simulink model "SecRwRtStLgrstInwdOtwdTrgtPosSelc"  (R2018b)
settings: Solver=FixedStepDiscrete  StartTime=0.0  StopTime=10.0  FixedStep=0.01  RelTol=1e-3
undefined symbols (not defined in the file or in its folder): KeSMSw4SAcsMd24SecRwRtStLegrstOtwdInwdPos_Val, KeSMSw4SAcsMd24SecRwRtStLegrstOtwdInwdPosMax_Val, KeSMSw4SAcsMd24SecRwRtStLegrstOtwdInwdPosMin_Val, KeSMSw4SAcsMd26SecRwRtStLegrstOtwdInwdPos_Val, KeSMSw4SAcsMd26SecRwRtStLegrstOtwdInwdPosMax_Val, KeSMSw4SAcsMd26SecRwRtStLegrstOtwdInwdPosMin_Val, KeSMSw4SLegrstCloseMdSecRwRtStLgrstOtwdInwdPos_Val, KeSMSw4SLegrstCloseMdSecRwRtStLgrstOtwdInwdPosMax_Val, KeSMSw4SLegrstCloseMdSecRwRtStLgrstOtwdInwdPosMin_Val, KeSMSw4SLegrstOpenMdSecRwRtStLgrstOtwdInwdPos_Val, KeSMSw4SLegrstOpenMdSecRwRtStLgrstOtwdInwdPosMax_Val, KeSMSw4SLegrstOpenMdSecRwRtStLgrstOtwdInwdPosMin_Val, KeSMSw4sLyingMDSecRwRtStLgrstOtwdInwdPos_160_Val, KeSMSw4sLyingMDSecRwRtStLgrstOtwdInwdPos_165_Val, KeSMSw4sLyingMDSecRwRtStLgrstOtwdInwdPos_170_Val, KeSMSw4sLyingMDSecRwRtStLgrstOtwdInwdPos_175_Val, KeSMSw4sLyingMDSecRwRtStLgrstOtwdInwdPos_180_Val, KeSMSw4sLyingMDSecRwRtStLgrstOtwdInwdPos_Below160_Val, KeSMSw4sLyingMDSecRwRtStLgrstOtwdInwdPos_Over180_Val, KeSMSw4sLyingMDSecRwRtStLgrstOtwdInwdPosMax_160_Val, KeSMSw4sLyingMDSecRwRtStLgrstOtwdInwdPosMax_165_Val, KeSMSw4sLyingMDSecRwRtStLgrstOtwdInwdPosMax_170_Val, KeSMSw4sLyingMDSecRwRtStLgrstOtwdInwdPosMax_175_Val, KeSMSw4sLyingMDSecRwRtStLgrstOtwdInwdPosMax_180_Val, KeSMSw4sLyingMDSecRwRtStLgrstOtwdInwdPosMax_Below160_Val, KeSMSw4sLyingMDSecRwRtStLgrstOtwdInwdPosMax_Over180_Val, KeSMSw4sLyingMDSecRwRtStLgrstOtwdInwdPosMin_160_Val, KeSMSw4sLyingMDSecRwRtStLgrstOtwdInwdPosMin_165_Val, KeSMSw4sLyingMDSecRwRtStLgrstOtwdInwdPosMin_170_Val, KeSMSw4sLyingMDSecRwRtStLgrstOtwdInwdPosMin_175_Val, KeSMSw4sLyingMDSecRwRtStLgrstOtwdInwdPosMin_180_Val, KeSMSw4sLyingMDSecRwRtStLgrstOtwdInwdPosMin_Below160_Val, KeSMSw4sLyingMDSecRwRtStLgrstOtwdInwdPosMin_Over180_Val, KeSMSw4sRecoveryMDSecRwRtStLgrstOtwdInwdPos_160_Val, KeSMSw4sRecoveryMDSecRwRtStLgrstOtwdInwdPos_165_Val, KeSMSw4sRecoveryMDSecRwRtStLgrstOtwdInwdPos_170_Val, KeSMSw4sRecoveryMDSecRwRtStLgrstOtwdInwdPos_175_Val, KeSMSw4sRecoveryMDSecRwRtStLgrstOtwdInwdPos_180_Val, KeSMSw4sRecoveryMDSecRwRtStLgrstOtwdInwdPos_Below160_Val, KeSMSw4sRecoveryMDSecRwRtStLgrstOtwdInwdPos_Over180_Val, KeSMSw4sRecoveryMDSecRwRtStLgrstOtwdInwdPosMax_160_Val, KeSMSw4sRecoveryMDSecRwRtStLgrstOtwdInwdPosMax_165_Val, KeSMSw4sRecoveryMDSecRwRtStLgrstOtwdInwdPosMax_170_Val, KeSMSw4sRecoveryMDSecRwRtStLgrstOtwdInwdPosMax_175_Val, KeSMSw4sRecoveryMDSecRwRtStLgrstOtwdInwdPosMax_180_Val, KeSMSw4sRecoveryMDSecRwRtStLgrstOtwdInwdPosMax_Below160_Val, KeSMSw4sRecoveryMDSecRwRtStLgrstOtwdInwdPosMax_Over180_Val, KeSMSw4sRecoveryMDSecRwRtStLgrstOtwdInwdPosMin_160_Val, KeSMSw4sRecoveryMDSecRwRtStLgrstOtwdInwdPosMin_165_Val, KeSMSw4sRecoveryMDSecRwRtStLgrstOtwdInwdPosMin_170_Val, KeSMSw4sRecoveryMDSecRwRtStLgrstOtwdInwdPosMin_175_Val, KeSMSw4sRecoveryMDSecRwRtStLgrstOtwdInwdPosMin_180_Val, KeSMSw4sRecoveryMDSecRwRtStLgrstOtwdInwdPosMin_Below160_Val, KeSMSw4sRecoveryMDSecRwRtStLgrstOtwdInwdPosMin_Over180_Val, KeSMSw4sVIPMDSecRwRtStLgrstOtwdInwdPos_160_Val, KeSMSw4sVIPMDSecRwRtStLgrstOtwdInwdPos_165_Val, KeSMSw4sVIPMDSecRwRtStLgrstOtwdInwdPos_170_Val, KeSMSw4sVIPMDSecRwRtStLgrstOtwdInwdPos_175_Val, KeSMSw4sVIPMDSecRwRtStLgrstOtwdInwdPos_180_Val, KeSMSw4sVIPMDSecRwRtStLgrstOtwdInwdPos_Below160_Val ... (+40)
libraries: TrgtPosSelcLib x10
(part 1 of 2)
settings Model: Creator=sn2xws  LastModifiedBy=sn2xws
settings Model: ModifiedHistory=|
  | 2023.8.1 V2.0.0 CR401790 增加模式21-26
  | 2024.5.6 V3.0.0 557 67座增加腿托延伸
  | 2024.7.9 V3.0.1557模式流程V1.9
settings DataIOCC: SaveFormat=StructureWithTime
settings OptimizationCC: DefaultParameterBehavior=Inlined  EnhancedBackFolding=on  PassReuseOutputArgsAs=Individual arguments  ZeroExternalMemoryAtStartup=off  ZeroInternalMemoryAtStartup=off  OptimizeBlockOrder=speed  DifferentSizesBufferReuse=on  OptimizationCustomize=off
settings DebuggingCC: ParameterTunabilityLossMsg=error
settings ModelReferenceCC: ModelReferenceNumInstancesAllowed=Single
settings SFSimCC: MATLABDynamicMemAlloc=off
settings RTWCC: SystemTargetFile=autosar.tlc  GenCodeOnly=on  TemplateMakefile=ert_default_tmf  Description=AUTOSAR  GenerateReport=on  IncludeHyperlinkInReport=on  LaunchReport=on  GenerateTraceInfo=on  GenerateTraceReport=on  GenerateTraceReportSl=on  GenerateTraceReportSf=on  GenerateTraceReportEml=on
settings CodeAppCC: ForceParamTrailComments=on  IgnoreCustomStorageClasses=off  OperatorAnnotations=on  SimulinkDataObjDesc=on  SFDataObjDesc=on  InsertBlockDesc=on
settings STFCustomTargetCC: TargetLangStandard=C99 (ISO)  MultiwordLength=256  ParMdlRefBuildCompliant=on  CompOptLevelCompliant=on  IncludeMdlTerminateFcn=off  CombineOutputUpdateFcns=on  SuppressErrorStatus=on  ERTCustomFileBanners=on  SupportNonFinite=off  SupportComplex=off  SupportContinuousTime=off  SupportNonInlinedSFcns=off  RemoveResetFunc=on  MATLABClassNameForMDSCustomization=Simulink.SoftwareTarget.ERTCustomization  AutosarCompliant=on  UseToolchainInfoCompliant=on  LookupTableObjectStructAxisOrder=2,1,3,4,...  LUTObjectStructOrderEvenSpacing=Size,Table,Breakpoints  SystemTargetFile=autosar.tlc
settings ERTTargetCC: TargetLangStandard=C99 (ISO)  ConcurrentExecutionCompliant=off  IncludeMdlTerminateFcn=off  SuppressErrorStatus=on  SupportNonFinite=off  SupportComplex=off  ModelStepFunctionPrototypeControlCompliant=off  CPPClassGenCompliant=off  AutosarCompliant=on  LookupTableObjectStructAxisOrder=2,1,3,4,...  LUTObjectStructOrderEvenSpacing=Size,Table,Breakpoints  InlinedParameterPlacement=NonHierarchical  ERTCustomFileTemplate=example_file_process.tlc  ERTFilePackagingFormat=Compact

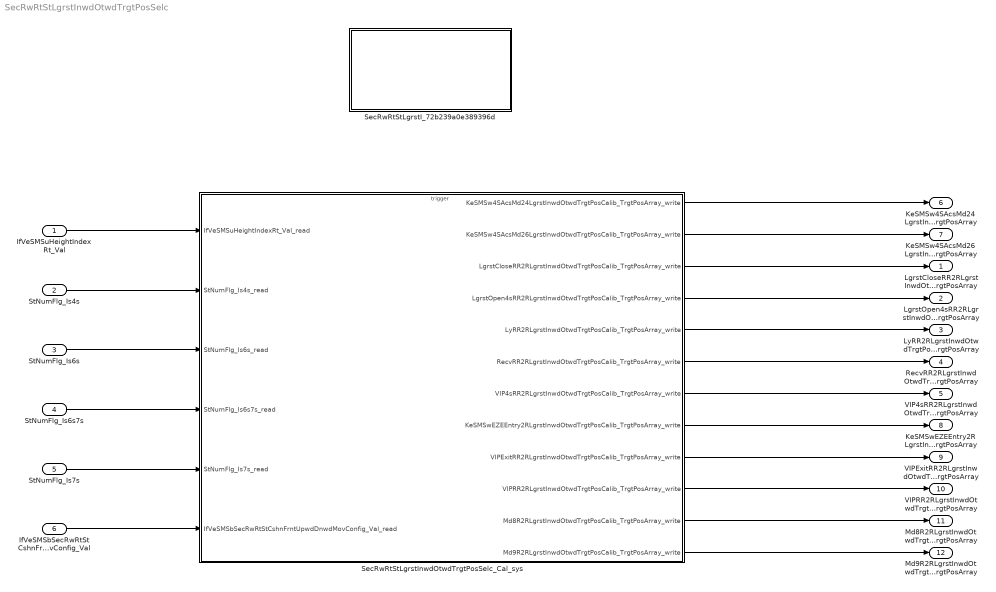
== system SecRwRtStLgrstInwdOtwdTrgtPosSelc ==
  IfVeSMSuHeightIndexRt_Val : Inport  Description=|  OutDataTypeStr=uint8  PortDimensions=1
      | 0：under 160
      | 1：160
      | 2：165
      | 3：170
      | 4：175
      | 5：180
      | 6：over 180
  StNumFlg_Is4s : Inport  Port=2  OutDataTypeStr=boolean  PortDimensions=1
  StNumFlg_Is6s : Inport  Port=3  OutDataTypeStr=boolean  PortDimensions=1
  StNumFlg_Is6s7s : Inport  Port=4  OutDataTypeStr=boolean  PortDimensions=1
  StNumFlg_Is7s : Inport  Port=5  OutDataTypeStr=boolean  PortDimensions=1
  IfVeSMSbSecRwRtStCshnFrntUpwdDnwdMovConfig_Val : Inport  Port=6  OutDataTypeStr=boolean  PortDimensions=1
  SecRwRtStLgrstI_72b239a0e389396d : Subsystem
  SecRwRtStLgrstInwdOtwdTrgtPosSelc_Cal_sys : Subsystem
  LgrstCloseRR2RLgrstInwdOtwdTrgtPosCalib_TrgtPosArray : Outport  Description=|  OutDataTypeStr=uint16  PortDimensions=3
      | 0:Pos
      | 1:Max
      | 2:Min
  LgrstOpen4sRR2RLgrstInwdOtwdTrgtPosCalib_TrgtPosArray : Outport  Description=|  Port=2  OutDataTypeStr=uint16  PortDimensions=3
      | 0:Pos
      | 1:Max
      | 2:Min
  LyRR2RLgrstInwdOtwdTrgtPosCalib_TrgtPosArray : Outport  Description=|  Port=3  OutDataTypeStr=uint16  PortDimensions=3
      | 0:Pos
      | 1:Max
      | 2:Min
  RecvRR2RLgrstInwdOtwdTrgtPosCalib_TrgtPosArray : Outport  Description=|  Port=4  OutDataTypeStr=uint16  PortDimensions=3
      | 0:Pos
      | 1:Max
      | 2:Min
  VIP4sRR2RLgrstInwdOtwdTrgtPosCalib_TrgtPosArray : Outport  Description=|  Port=5  OutDataTypeStr=uint16  PortDimensions=3
      | 0:Pos
      | 1:Max
      | 2:Min
  KeSMSw4SAcsMd24LgrstInwdOtwdTrgtPosCalib_TrgtPosArray : Outport  Description=|  Port=6  OutDataTypeStr=uint16  PortDimensions=3
      | 0:Pos
      | 1:Max
      | 2:Min
  KeSMSw4SAcsMd26LgrstInwdOtwdTrgtPosCalib_TrgtPosArray : Outport  Description=|  Port=7  OutDataTypeStr=uint16  PortDimensions=3
      | 0:Pos
      | 1:Max
      | 2:Min
  KeSMSwEZEEntry2RLgrstInwdOtwdTrgtPosCalib_TrgtPosArray : Outport  Description=|  Port=8  OutDataTypeStr=uint16  PortDimensions=3
      | 0:Pos
      | 1:Max
      | 2:Min
  VIPExitRR2RLgrstInwdOtwdTrgtPosCalib_TrgtPosArray : Outport  Description=|  Port=9  OutDataTypeStr=uint16  PortDimensions=3
      | 0:Pos
      | 1:Max
      | 2:Min
  VIPRR2RLgrstInwdOtwdTrgtPosCalib_TrgtPosArray : Outport  Description=|  Port=10  OutDataTypeStr=uint16  PortDimensions=3
      | 0:Pos
      | 1:Max
      | 2:Min
  Md8R2RLgrstInwdOtwdTrgtPosCalib_TrgtPosArray : Outport  Description=|  Port=11  OutDataTypeStr=uint16  PortDimensions=3
      | 0:Pos
      | 1:Max
      | 2:Min
  Md9R2RLgrstInwdOtwdTrgtPosCalib_TrgtPosArray : Outport  Description=|  Port=12  OutDataTypeStr=uint16  PortDimensions=3
      | 0:Pos
      | 1:Max
      | 2:Min
  wires:
  IfVeSMSuHeightIndexRt_Val/1 -> SecRwRtStLgrstInwdOtwdTrgtPosSelc_Cal_sys/1(IfVeSMSuHeightIndexRt_Val_read)
  StNumFlg_Is4s/1 -> SecRwRtStLgrstInwdOtwdTrgtPosSelc_Cal_sys/2(StNumFlg_Is4s_read)
  StNumFlg_Is6s/1 -> SecRwRtStLgrstInwdOtwdTrgtPosSelc_Cal_sys/3(StNumFlg_Is6s_read)
  StNumFlg_Is6s7s/1 -> SecRwRtStLgrstInwdOtwdTrgtPosSelc_Cal_sys/4(StNumFlg_Is6s7s_read)
  StNumFlg_Is7s/1 -> SecRwRtStLgrstInwdOtwdTrgtPosSelc_Cal_sys/5(StNumFlg_Is7s_read)
  SecRwRtStLgrstInwdOtwdTrgtPosSelc_Cal_sys/3(LgrstCloseRR2RLgrstInwdOtwdTrgtPosCalib_TrgtPosArray_write) -> LgrstCloseRR2RLgrstInwdOtwdTrgtPosCalib_TrgtPosArray/1
  SecRwRtStLgrstInwdOtwdTrgtPosSelc_Cal_sys/4(LgrstOpen4sRR2RLgrstInwdOtwdTrgtPosCalib_TrgtPosArray_write) -> LgrstOpen4sRR2RLgrstInwdOtwdTrgtPosCalib_TrgtPosArray/1
  SecRwRtStLgrstInwdOtwdTrgtPosSelc_Cal_sys/5(LyRR2RLgrstInwdOtwdTrgtPosCalib_TrgtPosArray_write) -> LyRR2RLgrstInwdOtwdTrgtPosCalib_TrgtPosArray/1
  SecRwRtStLgrstInwdOtwdTrgtPosSelc_Cal_sys/6(RecvRR2RLgrstInwdOtwdTrgtPosCalib_TrgtPosArray_write) -> RecvRR2RLgrstInwdOtwdTrgtPosCalib_TrgtPosArray/1
  SecRwRtStLgrstInwdOtwdTrgtPosSelc_Cal_sys/7(VIP4sRR2RLgrstInwdOtwdTrgtPosCalib_TrgtPosArray_write) -> VIP4sRR2RLgrstInwdOtwdTrgtPosCalib_TrgtPosArray/1
  SecRwRtStLgrstInwdOtwdTrgtPosSelc_Cal_sys/1(KeSMSw4SAcsMd24LgrstInwdOtwdTrgtPosCalib_TrgtPosArray_write) -> KeSMSw4SAcsMd24LgrstInwdOtwdTrgtPosCalib_TrgtPosArray/1
  SecRwRtStLgrstInwdOtwdTrgtPosSelc_Cal_sys/2(KeSMSw4SAcsMd26LgrstInwdOtwdTrgtPosCalib_TrgtPosArray_write) -> KeSMSw4SAcsMd26LgrstInwdOtwdTrgtPosCalib_TrgtPosArray/1
  SecRwRtStLgrstInwdOtwdTrgtPosSelc_Cal_sys/8(KeSMSwEZEEntry2RLgrstInwdOtwdTrgtPosCalib_TrgtPosArray_write) -> KeSMSwEZEEntry2RLgrstInwdOtwdTrgtPosCalib_TrgtPosArray/1
  IfVeSMSbSecRwRtStCshnFrntUpwdDnwdMovConfig_Val/1 -> SecRwRtStLgrstInwdOtwdTrgtPosSelc_Cal_sys/6(IfVeSMSbSecRwRtStCshnFrntUpwdDnwdMovConfig_Val_read)
  SecRwRtStLgrstInwdOtwdTrgtPosSelc_Cal_sys/9(VIPExitRR2RLgrstInwdOtwdTrgtPosCalib_TrgtPosArray_write) -> VIPExitRR2RLgrstInwdOtwdTrgtPosCalib_TrgtPosArray/1
  SecRwRtStLgrstInwdOtwdTrgtPosSelc_Cal_sys/10(VIPRR2RLgrstInwdOtwdTrgtPosCalib_TrgtPosArray_write) -> VIPRR2RLgrstInwdOtwdTrgtPosCalib_TrgtPosArray/1
  SecRwRtStLgrstInwdOtwdTrgtPosSelc_Cal_sys/11(Md8R2RLgrstInwdOtwdTrgtPosCalib_TrgtPosArray_write) -> Md8R2RLgrstInwdOtwdTrgtPosCalib_TrgtPosArray/1
  SecRwRtStLgrstInwdOtwdTrgtPosSelc_Cal_sys/12(Md9R2RLgrstInwdOtwdTrgtPosCalib_TrgtPosArray_write) -> Md9R2RLgrstInwdOtwdTrgtPosCalib_TrgtPosArray/1

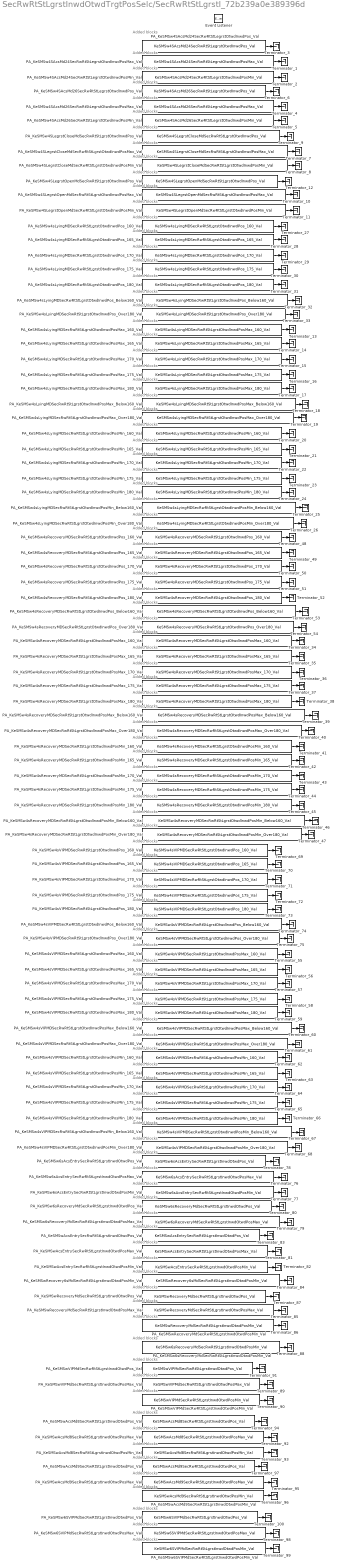
== system SecRwRtStLgrstInwdOtwdTrgtPosSelc/SecRwRtStLgrstI_72b239a0e389396d ==
  note: Added blocks
  note: Added blocks
  note: Added blocks
  note: Added blocks
  note: Added blocks
  note: Added blocks
  note: Added blocks
  note: Added blocks
  note: Added blocks
  note: Added blocks
  note: Added blocks
  note: Added blocks
  note: Added blocks
  note: Added blocks
  note: Added blocks
  note: Added blocks
  note: Added blocks
  note: Added blocks
  note: Added blocks
  note: Added blocks
  note: Added blocks
  note: Added blocks
  note: Added blocks
  note: Added blocks
  note: Added blocks
  note: Added blocks
  note: Added blocks
  note: Added blocks
  note: Added blocks
  note: Added blocks
  note: Added blocks
  note: Added blocks
  note: Added blocks
  note: Added blocks
  note: Added blocks
  note: Added blocks
  note: Added blocks
  note: Added blocks
  note: Added blocks
  note: Added blocks
  note: Added blocks
  note: Added blocks
  note: Added blocks
  note: Added blocks
  note: Added blocks
  note: Added blocks
  note: Added blocks
  note: Added blocks
  note: Added blocks
  note: Added blocks
  note: Added blocks
  note: Added blocks
  note: Added blocks
  note: Added blocks
  note: Added blocks
  note: Added blocks
  note: Added blocks
  note: Added blocks
  note: Added blocks
  note: Added blocks
  note: Added blocks
  note: Added blocks
  note: Added blocks
  note: Added blocks
  note: Added blocks
  note: Added blocks
  note: Added blocks
  note: Added blocks
  note: Added blocks
  note: Added blocks
  note: Added blocks
  note: Added blocks
  note: Added blocks
  note: Added blocks
  note: Added blocks
  note: Added blocks
  note: Added blocks
  note: Added blocks
  note: Added blocks
  note: Added blocks
  note: Added blocks
  note: Added blocks
  note: Added blocks
  note: Added blocks
  note: Added blocks
  note: Added blocks
  note: Added blocks
  note: Added blocks
  note: Added blocks
  note: Added blocks
  note: Added blocks
  note: Added blocks
  note: Added blocks
  note: Added blocks
  note: Added blocks
  note: Added blocks
  note: Added blocks
  note: Added blocks
  note: Added blocks
  note: Added blocks
  Event Listener : EventListener  EventName=reset
  PA_KeSMSw4SAcsMd24SecRwRtStLegrstOtwdInwdPosMax_Val : Constant  Value=KeSMSw4SAcsMd24SecRwRtStLegrstOtwdInwdPosMax_Val
  PA_KeSMSw4SAcsMd24SecRwRtStLegrstOtwdInwdPosMin_Val : Constant  Value=KeSMSw4SAcsMd24SecRwRtStLegrstOtwdInwdPosMin_Val
  PA_KeSMSw4SAcsMd24SecRwRtStLegrstOtwdInwdPos_Val : Constant  Value=KeSMSw4SAcsMd24SecRwRtStLegrstOtwdInwdPos_Val
  PA_KeSMSw4SAcsMd26SecRwRtStLegrstOtwdInwdPosMax_Val : Constant  Value=KeSMSw4SAcsMd26SecRwRtStLegrstOtwdInwdPosMax_Val
  PA_KeSMSw4SAcsMd26SecRwRtStLegrstOtwdInwdPosMin_Val : Constant  Value=KeSMSw4SAcsMd26SecRwRtStLegrstOtwdInwdPosMin_Val
  PA_KeSMSw4SAcsMd26SecRwRtStLegrstOtwdInwdPos_Val : Constant  Value=KeSMSw4SAcsMd26SecRwRtStLegrstOtwdInwdPos_Val
  PA_KeSMSw4SLegrstCloseMdSecRwRtStLgrstOtwdInwdPosMax_Val : Constant  Value=KeSMSw4SLegrstCloseMdSecRwRtStLgrstOtwdInwdPosMax_Val
  PA_KeSMSw4SLegrstCloseMdSecRwRtStLgrstOtwdInwdPosMin_Val : Constant  Value=KeSMSw4SLegrstCloseMdSecRwRtStLgrstOtwdInwdPosMin_Val
  PA_KeSMSw4SLegrstCloseMdSecRwRtStLgrstOtwdInwdPos_Val : Constant  Value=KeSMSw4SLegrstCloseMdSecRwRtStLgrstOtwdInwdPos_Val
  PA_KeSMSw4SLegrstOpenMdSecRwRtStLgrstOtwdInwdPosMax_Val : Constant  Value=KeSMSw4SLegrstOpenMdSecRwRtStLgrstOtwdInwdPosMax_Val
  PA_KeSMSw4SLegrstOpenMdSecRwRtStLgrstOtwdInwdPosMin_Val : Constant  Value=KeSMSw4SLegrstOpenMdSecRwRtStLgrstOtwdInwdPosMin_Val
  PA_KeSMSw4SLegrstOpenMdSecRwRtStLgrstOtwdInwdPos_Val : Constant  Value=KeSMSw4SLegrstOpenMdSecRwRtStLgrstOtwdInwdPos_Val
  PA_KeSMSw4sLyingMDSecRwRtStLgrstOtwdInwdPosMax_160_Val : Constant  Value=KeSMSw4sLyingMDSecRwRtStLgrstOtwdInwdPosMax_160_Val
  PA_KeSMSw4sLyingMDSecRwRtStLgrstOtwdInwdPosMax_165_Val : Constant  Value=KeSMSw4sLyingMDSecRwRtStLgrstOtwdInwdPosMax_165_Val
  PA_KeSMSw4sLyingMDSecRwRtStLgrstOtwdInwdPosMax_170_Val : Constant  Value=KeSMSw4sLyingMDSecRwRtStLgrstOtwdInwdPosMax_170_Val
  PA_KeSMSw4sLyingMDSecRwRtStLgrstOtwdInwdPosMax_175_Val : Constant  Value=KeSMSw4sLyingMDSecRwRtStLgrstOtwdInwdPosMax_175_Val
  PA_KeSMSw4sLyingMDSecRwRtStLgrstOtwdInwdPosMax_180_Val : Constant  Value=KeSMSw4sLyingMDSecRwRtStLgrstOtwdInwdPosMax_180_Val
  PA_KeSMSw4sLyingMDSecRwRtStLgrstOtwdInwdPosMax_Below160_Val : Constant  Value=KeSMSw4sLyingMDSecRwRtStLgrstOtwdInwdPosMax_Below160_Val
  PA_KeSMSw4sLyingMDSecRwRtStLgrstOtwdInwdPosMax_Over180_Val : Constant  Value=KeSMSw4sLyingMDSecRwRtStLgrstOtwdInwdPosMax_Over180_Val
  PA_KeSMSw4sLyingMDSecRwRtStLgrstOtwdInwdPosMin_160_Val : Constant  Value=KeSMSw4sLyingMDSecRwRtStLgrstOtwdInwdPosMin_160_Val
  PA_KeSMSw4sLyingMDSecRwRtStLgrstOtwdInwdPosMin_165_Val : Constant  Value=KeSMSw4sLyingMDSecRwRtStLgrstOtwdInwdPosMin_165_Val
  PA_KeSMSw4sLyingMDSecRwRtStLgrstOtwdInwdPosMin_170_Val : Constant  Value=KeSMSw4sLyingMDSecRwRtStLgrstOtwdInwdPosMin_170_Val
  PA_KeSMSw4sLyingMDSecRwRtStLgrstOtwdInwdPosMin_175_Val : Constant  Value=KeSMSw4sLyingMDSecRwRtStLgrstOtwdInwdPosMin_175_Val
  PA_KeSMSw4sLyingMDSecRwRtStLgrstOtwdInwdPosMin_180_Val : Constant  Value=KeSMSw4sLyingMDSecRwRtStLgrstOtwdInwdPosMin_180_Val
  PA_KeSMSw4sLyingMDSecRwRtStLgrstOtwdInwdPosMin_Below160_Val : Constant  Value=KeSMSw4sLyingMDSecRwRtStLgrstOtwdInwdPosMin_Below160_Val
  PA_KeSMSw4sLyingMDSecRwRtStLgrstOtwdInwdPosMin_Over180_Val : Constant  Value=KeSMSw4sLyingMDSecRwRtStLgrstOtwdInwdPosMin_Over180_Val
  PA_KeSMSw4sLyingMDSecRwRtStLgrstOtwdInwdPos_160_Val : Constant  Value=KeSMSw4sLyingMDSecRwRtStLgrstOtwdInwdPos_160_Val
  PA_KeSMSw4sLyingMDSecRwRtStLgrstOtwdInwdPos_165_Val : Constant  Value=KeSMSw4sLyingMDSecRwRtStLgrstOtwdInwdPos_165_Val
  PA_KeSMSw4sLyingMDSecRwRtStLgrstOtwdInwdPos_170_Val : Constant  Value=KeSMSw4sLyingMDSecRwRtStLgrstOtwdInwdPos_170_Val
  PA_KeSMSw4sLyingMDSecRwRtStLgrstOtwdInwdPos_175_Val : Constant  Value=KeSMSw4sLyingMDSecRwRtStLgrstOtwdInwdPos_175_Val
  PA_KeSMSw4sLyingMDSecRwRtStLgrstOtwdInwdPos_180_Val : Constant  Value=KeSMSw4sLyingMDSecRwRtStLgrstOtwdInwdPos_180_Val
  PA_KeSMSw4sLyingMDSecRwRtStLgrstOtwdInwdPos_Below160_Val : Constant  Value=KeSMSw4sLyingMDSecRwRtStLgrstOtwdInwdPos_Below160_Val
  PA_KeSMSw4sLyingMDSecRwRtStLgrstOtwdInwdPos_Over180_Val : Constant  Value=KeSMSw4sLyingMDSecRwRtStLgrstOtwdInwdPos_Over180_Val
  PA_KeSMSw4sRecoveryMDSecRwRtStLgrstOtwdInwdPosMax_160_Val : Constant  Value=KeSMSw4sRecoveryMDSecRwRtStLgrstOtwdInwdPosMax_160_Val
  PA_KeSMSw4sRecoveryMDSecRwRtStLgrstOtwdInwdPosMax_165_Val : Constant  Value=KeSMSw4sRecoveryMDSecRwRtStLgrstOtwdInwdPosMax_165_Val
  PA_KeSMSw4sRecoveryMDSecRwRtStLgrstOtwdInwdPosMax_170_Val : Constant  Value=KeSMSw4sRecoveryMDSecRwRtStLgrstOtwdInwdPosMax_170_Val
  PA_KeSMSw4sRecoveryMDSecRwRtStLgrstOtwdInwdPosMax_175_Val : Constant  Value=KeSMSw4sRecoveryMDSecRwRtStLgrstOtwdInwdPosMax_175_Val
  PA_KeSMSw4sRecoveryMDSecRwRtStLgrstOtwdInwdPosMax_180_Val : Constant  Value=KeSMSw4sRecoveryMDSecRwRtStLgrstOtwdInwdPosMax_180_Val
  PA_KeSMSw4sRecoveryMDSecRwRtStLgrstOtwdInwdPosMax_Below160_Val : Constant  Value=KeSMSw4sRecoveryMDSecRwRtStLgrstOtwdInwdPosMax_Below160_Val
  PA_KeSMSw4sRecoveryMDSecRwRtStLgrstOtwdInwdPosMax_Over180_Val : Constant  Value=KeSMSw4sRecoveryMDSecRwRtStLgrstOtwdInwdPosMax_Over180_Val
  PA_KeSMSw4sRecoveryMDSecRwRtStLgrstOtwdInwdPosMin_160_Val : Constant  Value=KeSMSw4sRecoveryMDSecRwRtStLgrstOtwdInwdPosMin_160_Val
  PA_KeSMSw4sRecoveryMDSecRwRtStLgrstOtwdInwdPosMin_165_Val : Constant  Value=KeSMSw4sRecoveryMDSecRwRtStLgrstOtwdInwdPosMin_165_Val
  PA_KeSMSw4sRecoveryMDSecRwRtStLgrstOtwdInwdPosMin_170_Val : Constant  Value=KeSMSw4sRecoveryMDSecRwRtStLgrstOtwdInwdPosMin_170_Val
  PA_KeSMSw4sRecoveryMDSecRwRtStLgrstOtwdInwdPosMin_175_Val : Constant  Value=KeSMSw4sRecoveryMDSecRwRtStLgrstOtwdInwdPosMin_175_Val
  PA_KeSMSw4sRecoveryMDSecRwRtStLgrstOtwdInwdPosMin_180_Val : Constant  Value=KeSMSw4sRecoveryMDSecRwRtStLgrstOtwdInwdPosMin_180_Val
  PA_KeSMSw4sRecoveryMDSecRwRtStLgrstOtwdInwdPosMin_Below160_Val : Constant  Value=KeSMSw4sRecoveryMDSecRwRtStLgrstOtwdInwdPosMin_Below160_Val
  PA_KeSMSw4sRecoveryMDSecRwRtStLgrstOtwdInwdPosMin_Over180_Val : Constant  Value=KeSMSw4sRecoveryMDSecRwRtStLgrstOtwdInwdPosMin_Over180_Val
  PA_KeSMSw4sRecoveryMDSecRwRtStLgrstOtwdInwdPos_160_Val : Constant  Value=KeSMSw4sRecoveryMDSecRwRtStLgrstOtwdInwdPos_160_Val
  PA_KeSMSw4sRecoveryMDSecRwRtStLgrstOtwdInwdPos_165_Val : Constant  Value=KeSMSw4sRecoveryMDSecRwRtStLgrstOtwdInwdPos_165_Val
  PA_KeSMSw4sRecoveryMDSecRwRtStLgrstOtwdInwdPos_170_Val : Constant  Value=KeSMSw4sRecoveryMDSecRwRtStLgrstOtwdInwdPos_170_Val
  PA_KeSMSw4sRecoveryMDSecRwRtStLgrstOtwdInwdPos_175_Val : Constant  Value=KeSMSw4sRecoveryMDSecRwRtStLgrstOtwdInwdPos_175_Val
  PA_KeSMSw4sRecoveryMDSecRwRtStLgrstOtwdInwdPos_180_Val : Constant  Value=KeSMSw4sRecoveryMDSecRwRtStLgrstOtwdInwdPos_180_Val
  PA_KeSMSw4sRecoveryMDSecRwRtStLgrstOtwdInwdPos_Below160_Val : Constant  Value=KeSMSw4sRecoveryMDSecRwRtStLgrstOtwdInwdPos_Below160_Val
  PA_KeSMSw4sRecoveryMDSecRwRtStLgrstOtwdInwdPos_Over180_Val : Constant  Value=KeSMSw4sRecoveryMDSecRwRtStLgrstOtwdInwdPos_Over180_Val
  PA_KeSMSw4sVIPMDSecRwRtStLgrstOtwdInwdPosMax_160_Val : Constant  Value=KeSMSw4sVIPMDSecRwRtStLgrstOtwdInwdPosMax_160_Val
  PA_KeSMSw4sVIPMDSecRwRtStLgrstOtwdInwdPosMax_165_Val : Constant  Value=KeSMSw4sVIPMDSecRwRtStLgrstOtwdInwdPosMax_165_Val
  PA_KeSMSw4sVIPMDSecRwRtStLgrstOtwdInwdPosMax_170_Val : Constant  Value=KeSMSw4sVIPMDSecRwRtStLgrstOtwdInwdPosMax_170_Val
  PA_KeSMSw4sVIPMDSecRwRtStLgrstOtwdInwdPosMax_175_Val : Constant  Value=KeSMSw4sVIPMDSecRwRtStLgrstOtwdInwdPosMax_175_Val
  PA_KeSMSw4sVIPMDSecRwRtStLgrstOtwdInwdPosMax_180_Val : Constant  Value=KeSMSw4sVIPMDSecRwRtStLgrstOtwdInwdPosMax_180_Val
  PA_KeSMSw4sVIPMDSecRwRtStLgrstOtwdInwdPosMax_Below160_Val : Constant  Value=KeSMSw4sVIPMDSecRwRtStLgrstOtwdInwdPosMax_Below160_Val
  PA_KeSMSw4sVIPMDSecRwRtStLgrstOtwdInwdPosMax_Over180_Val : Constant  Value=KeSMSw4sVIPMDSecRwRtStLgrstOtwdInwdPosMax_Over180_Val
  PA_KeSMSw4sVIPMDSecRwRtStLgrstOtwdInwdPosMin_160_Val : Constant  Value=KeSMSw4sVIPMDSecRwRtStLgrstOtwdInwdPosMin_160_Val
  PA_KeSMSw4sVIPMDSecRwRtStLgrstOtwdInwdPosMin_165_Val : Constant  Value=KeSMSw4sVIPMDSecRwRtStLgrstOtwdInwdPosMin_165_Val
  PA_KeSMSw4sVIPMDSecRwRtStLgrstOtwdInwdPosMin_170_Val : Constant  Value=KeSMSw4sVIPMDSecRwRtStLgrstOtwdInwdPosMin_170_Val
  PA_KeSMSw4sVIPMDSecRwRtStLgrstOtwdInwdPosMin_175_Val : Constant  Value=KeSMSw4sVIPMDSecRwRtStLgrstOtwdInwdPosMin_175_Val
  PA_KeSMSw4sVIPMDSecRwRtStLgrstOtwdInwdPosMin_180_Val : Constant  Value=KeSMSw4sVIPMDSecRwRtStLgrstOtwdInwdPosMin_180_Val
  PA_KeSMSw4sVIPMDSecRwRtStLgrstOtwdInwdPosMin_Below160_Val : Constant  Value=KeSMSw4sVIPMDSecRwRtStLgrstOtwdInwdPosMin_Below160_Val
  PA_KeSMSw4sVIPMDSecRwRtStLgrstOtwdInwdPosMin_Over180_Val : Constant  Value=KeSMSw4sVIPMDSecRwRtStLgrstOtwdInwdPosMin_Over180_Val
  PA_KeSMSw4sVIPMDSecRwRtStLgrstOtwdInwdPos_160_Val : Constant  Value=KeSMSw4sVIPMDSecRwRtStLgrstOtwdInwdPos_160_Val
  PA_KeSMSw4sVIPMDSecRwRtStLgrstOtwdInwdPos_165_Val : Constant  Value=KeSMSw4sVIPMDSecRwRtStLgrstOtwdInwdPos_165_Val
  PA_KeSMSw4sVIPMDSecRwRtStLgrstOtwdInwdPos_170_Val : Constant  Value=KeSMSw4sVIPMDSecRwRtStLgrstOtwdInwdPos_170_Val
  PA_KeSMSw4sVIPMDSecRwRtStLgrstOtwdInwdPos_175_Val : Constant  Value=KeSMSw4sVIPMDSecRwRtStLgrstOtwdInwdPos_175_Val
  PA_KeSMSw4sVIPMDSecRwRtStLgrstOtwdInwdPos_180_Val : Constant  Value=KeSMSw4sVIPMDSecRwRtStLgrstOtwdInwdPos_180_Val
  PA_KeSMSw4sVIPMDSecRwRtStLgrstOtwdInwdPos_Below160_Val : Constant  Value=KeSMSw4sVIPMDSecRwRtStLgrstOtwdInwdPos_Below160_Val
  PA_KeSMSw4sVIPMDSecRwRtStLgrstOtwdInwdPos_Over180_Val : Constant  Value=KeSMSw4sVIPMDSecRwRtStLgrstOtwdInwdPos_Over180_Val
  PA_KeSMSw6SVIPMdSecRwRtStLgrstInwdOtwdPosMax_Val : Constant  Value=KeSMSw6SVIPMdSecRwRtStLgrstInwdOtwdPosMax_Val
  PA_KeSMSw6SVIPMdSecRwRtStLgrstInwdOtwdPosMin_Val : Constant  Value=KeSMSw6SVIPMdSecRwRtStLgrstInwdOtwdPosMin_Val
  PA_KeSMSw6SVIPMdSecRwRtStLgrstInwdOtwdPos_Val : Constant  Value=KeSMSw6SVIPMdSecRwRtStLgrstInwdOtwdPos_Val
  PA_KeSMSw6sAcsEntrySecRwRtStLgrstInwdOtwdPosMax_Val : Constant  Value=KeSMSw6sAcsEntrySecRwRtStLgrstInwdOtwdPosMax_Val
  PA_KeSMSw6sAcsEntrySecRwRtStLgrstInwdOtwdPosMin_Val : Constant  Value=KeSMSw6sAcsEntrySecRwRtStLgrstInwdOtwdPosMin_Val
  PA_KeSMSw6sAcsEntrySecRwRtStLgrstInwdOtwdPos_Val : Constant  Value=KeSMSw6sAcsEntrySecRwRtStLgrstInwdOtwdPos_Val
  PA_KeSMSw6sRecoveryMdSecRwRtStLgrstInwdOtwdPosMax_Val : Constant  Value=KeSMSw6sRecoveryMdSecRwRtStLgrstInwdOtwdPosMax_Val
  PA_KeSMSw6sRecoveryMdSecRwRtStLgrstInwdOtwdPosMin_Val : Constant  Value=KeSMSw6sRecoveryMdSecRwRtStLgrstInwdOtwdPosMin_Val
  PA_KeSMSw6sRecoveryMdSecRwRtStLgrstInwdOtwdPos_Val : Constant  Value=KeSMSw6sRecoveryMdSecRwRtStLgrstInwdOtwdPos_Val
  PA_KeSMSwAcsEntrySecRwRtStLgrstInwdOtwdPosMax_Val : Constant  Value=KeSMSwAcsEntrySecRwRtStLgrstInwdOtwdPosMax_Val
  PA_KeSMSwAcsEntrySecRwRtStLgrstInwdOtwdPosMin_Val : Constant  Value=KeSMSwAcsEntrySecRwRtStLgrstInwdOtwdPosMin_Val
  PA_KeSMSwAcsEntrySecRwRtStLgrstInwdOtwdPos_Val : Constant  Value=KeSMSwAcsEntrySecRwRtStLgrstInwdOtwdPos_Val
  PA_KeSMSwAcsMd8SecRwRtStLgrstInwdOtwdPosMax_Val : Constant  Value=KeSMSwAcsMd8SecRwRtStLgrstInwdOtwdPosMax_Val
  PA_KeSMSwAcsMd8SecRwRtStLgrstInwdOtwdPosMin_Val : Constant  Value=KeSMSwAcsMd8SecRwRtStLgrstInwdOtwdPosMin_Val
  PA_KeSMSwAcsMd8SecRwRtStLgrstInwdOtwdPos_Val : Constant  Value=KeSMSwAcsMd8SecRwRtStLgrstInwdOtwdPos_Val
  PA_KeSMSwAcsMd9SecRwRtStLgrstInwdOtwdPosMax_Val : Constant  Value=KeSMSwAcsMd9SecRwRtStLgrstInwdOtwdPosMax_Val
  PA_KeSMSwAcsMd9SecRwRtStLgrstInwdOtwdPosMin_Val : Constant  Value=KeSMSwAcsMd9SecRwRtStLgrstInwdOtwdPosMin_Val
  PA_KeSMSwAcsMd9SecRwRtStLgrstInwdOtwdPos_Val : Constant  Value=KeSMSwAcsMd9SecRwRtStLgrstInwdOtwdPos_Val
  PA_KeSMSwRecovery6sMdSecRwRtStLgrstInwdOtwdPosMin_Val : Constant  Value=KeSMSwRecovery6sMdSecRwRtStLgrstInwdOtwdPosMin_Val
  PA_KeSMSwRecoveryMdSecRwRtStLgrstInwdOtwdPosMax_Val : Constant  Value=KeSMSwRecoveryMdSecRwRtStLgrstInwdOtwdPosMax_Val
  PA_KeSMSwRecoveryMdSecRwRtStLgrstInwdOtwdPosMin_Val : Constant  Value=KeSMSwRecoveryMdSecRwRtStLgrstInwdOtwdPosMin_Val
  PA_KeSMSwRecoveryMdSecRwRtStLgrstInwdOtwdPos_Val : Constant  Value=KeSMSwRecoveryMdSecRwRtStLgrstInwdOtwdPos_Val
  PA_KeSMSwVIPMdSecRwRtStLgrstInwdOtwdPosMax_Val : Constant  Value=KeSMSwVIPMdSecRwRtStLgrstInwdOtwdPosMax_Val
  PA_KeSMSwVIPMdSecRwRtStLgrstInwdOtwdPosMin_Val : Constant  Value=KeSMSwVIPMdSecRwRtStLgrstInwdOtwdPosMin_Val
  PA_KeSMSwVIPMdSecRwRtStLgrstInwdOtwdPos_Val : Constant  Value=KeSMSwVIPMdSecRwRtStLgrstInwdOtwdPos_Val
  Terminator_{1..100} (100 alike) : Terminator
  wires:
  PA_KeSMSw4SAcsMd24SecRwRtStLegrstOtwdInwdPosMax_Val/1 -> Terminator_1/1
  PA_KeSMSw4SAcsMd24SecRwRtStLegrstOtwdInwdPosMin_Val/1 -> Terminator_2/1
  PA_KeSMSw4SAcsMd24SecRwRtStLegrstOtwdInwdPos_Val/1 -> Terminator_3/1
  PA_KeSMSw4SAcsMd26SecRwRtStLegrstOtwdInwdPosMax_Val/1 -> Terminator_4/1
  PA_KeSMSw4SAcsMd26SecRwRtStLegrstOtwdInwdPosMin_Val/1 -> Terminator_5/1
  PA_KeSMSw4SAcsMd26SecRwRtStLegrstOtwdInwdPos_Val/1 -> Terminator_6/1
  PA_KeSMSw4SLegrstCloseMdSecRwRtStLgrstOtwdInwdPosMax_Val/1 -> Terminator_7/1
  PA_KeSMSw4SLegrstCloseMdSecRwRtStLgrstOtwdInwdPosMin_Val/1 -> Terminator_8/1
  PA_KeSMSw4SLegrstCloseMdSecRwRtStLgrstOtwdInwdPos_Val/1 -> Terminator_9/1
  PA_KeSMSw4SLegrstOpenMdSecRwRtStLgrstOtwdInwdPosMax_Val/1 -> Terminator_10/1
  PA_KeSMSw4SLegrstOpenMdSecRwRtStLgrstOtwdInwdPosMin_Val/1 -> Terminator_11/1
  PA_KeSMSw4SLegrstOpenMdSecRwRtStLgrstOtwdInwdPos_Val/1 -> Terminator_12/1
  PA_KeSMSw4sLyingMDSecRwRtStLgrstOtwdInwdPosMax_160_Val/1 -> Terminator_13/1
  PA_KeSMSw4sLyingMDSecRwRtStLgrstOtwdInwdPosMax_165_Val/1 -> Terminator_14/1
  PA_KeSMSw4sLyingMDSecRwRtStLgrstOtwdInwdPosMax_170_Val/1 -> Terminator_15/1
  PA_KeSMSw4sLyingMDSecRwRtStLgrstOtwdInwdPosMax_175_Val/1 -> Terminator_16/1
  PA_KeSMSw4sLyingMDSecRwRtStLgrstOtwdInwdPosMax_180_Val/1 -> Terminator_17/1
  PA_KeSMSw4sLyingMDSecRwRtStLgrstOtwdInwdPosMax_Below160_Val/1 -> Terminator_18/1
  PA_KeSMSw4sLyingMDSecRwRtStLgrstOtwdInwdPosMax_Over180_Val/1 -> Terminator_19/1
  PA_KeSMSw4sLyingMDSecRwRtStLgrstOtwdInwdPosMin_160_Val/1 -> Terminator_20/1
  PA_KeSMSw4sLyingMDSecRwRtStLgrstOtwdInwdPosMin_165_Val/1 -> Terminator_21/1
  PA_KeSMSw4sLyingMDSecRwRtStLgrstOtwdInwdPosMin_170_Val/1 -> Terminator_22/1
  PA_KeSMSw4sLyingMDSecRwRtStLgrstOtwdInwdPosMin_175_Val/1 -> Terminator_23/1
  PA_KeSMSw4sLyingMDSecRwRtStLgrstOtwdInwdPosMin_180_Val/1 -> Terminator_24/1
  PA_KeSMSw4sLyingMDSecRwRtStLgrstOtwdInwdPosMin_Below160_Val/1 -> Terminator_25/1
  PA_KeSMSw4sLyingMDSecRwRtStLgrstOtwdInwdPosMin_Over180_Val/1 -> Terminator_26/1
  PA_KeSMSw4sLyingMDSecRwRtStLgrstOtwdInwdPos_160_Val/1 -> Terminator_27/1
  PA_KeSMSw4sLyingMDSecRwRtStLgrstOtwdInwdPos_165_Val/1 -> Terminator_28/1
  PA_KeSMSw4sLyingMDSecRwRtStLgrstOtwdInwdPos_170_Val/1 -> Terminator_29/1
  PA_KeSMSw4sLyingMDSecRwRtStLgrstOtwdInwdPos_175_Val/1 -> Terminator_30/1
  PA_KeSMSw4sLyingMDSecRwRtStLgrstOtwdInwdPos_180_Val/1 -> Terminator_31/1
  PA_KeSMSw4sLyingMDSecRwRtStLgrstOtwdInwdPos_Below160_Val/1 -> Terminator_32/1
  PA_KeSMSw4sLyingMDSecRwRtStLgrstOtwdInwdPos_Over180_Val/1 -> Terminator_33/1
  PA_KeSMSw4sRecoveryMDSecRwRtStLgrstOtwdInwdPosMax_160_Val/1 -> Terminator_34/1
  PA_KeSMSw4sRecoveryMDSecRwRtStLgrstOtwdInwdPosMax_165_Val/1 -> Terminator_35/1
  PA_KeSMSw4sRecoveryMDSecRwRtStLgrstOtwdInwdPosMax_170_Val/1 -> Terminator_36/1
  PA_KeSMSw4sRecoveryMDSecRwRtStLgrstOtwdInwdPosMax_175_Val/1 -> Terminator_37/1
  PA_KeSMSw4sRecoveryMDSecRwRtStLgrstOtwdInwdPosMax_180_Val/1 -> Terminator_38/1
  PA_KeSMSw4sRecoveryMDSecRwRtStLgrstOtwdInwdPosMax_Below160_Val/1 -> Terminator_39/1
  PA_KeSMSw4sRecoveryMDSecRwRtStLgrstOtwdInwdPosMax_Over180_Val/1 -> Terminator_40/1
  PA_KeSMSw4sRecoveryMDSecRwRtStLgrstOtwdInwdPosMin_160_Val/1 -> Terminator_41/1
  PA_KeSMSw4sRecoveryMDSecRwRtStLgrstOtwdInwdPosMin_165_Val/1 -> Terminator_42/1
  PA_KeSMSw4sRecoveryMDSecRwRtStLgrstOtwdInwdPosMin_170_Val/1 -> Terminator_43/1
  PA_KeSMSw4sRecoveryMDSecRwRtStLgrstOtwdInwdPosMin_175_Val/1 -> Terminator_44/1
  PA_KeSMSw4sRecoveryMDSecRwRtStLgrstOtwdInwdPosMin_180_Val/1 -> Terminator_45/1
  PA_KeSMSw4sRecoveryMDSecRwRtStLgrstOtwdInwdPosMin_Below160_Val/1 -> Terminator_46/1
  PA_KeSMSw4sRecoveryMDSecRwRtStLgrstOtwdInwdPosMin_Over180_Val/1 -> Terminator_47/1
  PA_KeSMSw4sRecoveryMDSecRwRtStLgrstOtwdInwdPos_160_Val/1 -> Terminator_48/1
  PA_KeSMSw4sRecoveryMDSecRwRtStLgrstOtwdInwdPos_165_Val/1 -> Terminator_49/1
  PA_KeSMSw4sRecoveryMDSecRwRtStLgrstOtwdInwdPos_170_Val/1 -> Terminator_50/1
  PA_KeSMSw4sRecoveryMDSecRwRtStLgrstOtwdInwdPos_175_Val/1 -> Terminator_51/1
  PA_KeSMSw4sRecoveryMDSecRwRtStLgrstOtwdInwdPos_180_Val/1 -> Terminator_52/1
  PA_KeSMSw4sRecoveryMDSecRwRtStLgrstOtwdInwdPos_Below160_Val/1 -> Terminator_53/1
  PA_KeSMSw4sRecoveryMDSecRwRtStLgrstOtwdInwdPos_Over180_Val/1 -> Terminator_54/1
  PA_KeSMSw4sVIPMDSecRwRtStLgrstOtwdInwdPosMax_160_Val/1 -> Terminator_55/1
  PA_KeSMSw4sVIPMDSecRwRtStLgrstOtwdInwdPosMax_165_Val/1 -> Terminator_56/1
  PA_KeSMSw4sVIPMDSecRwRtStLgrstOtwdInwdPosMax_170_Val/1 -> Terminator_57/1
  PA_KeSMSw4sVIPMDSecRwRtStLgrstOtwdInwdPosMax_175_Val/1 -> Terminator_58/1
  PA_KeSMSw4sVIPMDSecRwRtStLgrstOtwdInwdPosMax_180_Val/1 -> Terminator_59/1
  PA_KeSMSw4sVIPMDSecRwRtStLgrstOtwdInwdPosMax_Below160_Val/1 -> Terminator_60/1
  PA_KeSMSw4sVIPMDSecRwRtStLgrstOtwdInwdPosMax_Over180_Val/1 -> Terminator_61/1
  PA_KeSMSw4sVIPMDSecRwRtStLgrstOtwdInwdPosMin_160_Val/1 -> Terminator_62/1
  PA_KeSMSw4sVIPMDSecRwRtStLgrstOtwdInwdPosMin_165_Val/1 -> Terminator_63/1
  PA_KeSMSw4sVIPMDSecRwRtStLgrstOtwdInwdPosMin_170_Val/1 -> Terminator_64/1
  PA_KeSMSw4sVIPMDSecRwRtStLgrstOtwdInwdPosMin_175_Val/1 -> Terminator_65/1
  PA_KeSMSw4sVIPMDSecRwRtStLgrstOtwdInwdPosMin_180_Val/1 -> Terminator_66/1
  PA_KeSMSw4sVIPMDSecRwRtStLgrstOtwdInwdPosMin_Below160_Val/1 -> Terminator_67/1
  PA_KeSMSw4sVIPMDSecRwRtStLgrstOtwdInwdPosMin_Over180_Val/1 -> Terminator_68/1
  PA_KeSMSw4sVIPMDSecRwRtStLgrstOtwdInwdPos_160_Val/1 -> Terminator_69/1
  PA_KeSMSw4sVIPMDSecRwRtStLgrstOtwdInwdPos_165_Val/1 -> Terminator_70/1
  PA_KeSMSw4sVIPMDSecRwRtStLgrstOtwdInwdPos_170_Val/1 -> Terminator_71/1
  PA_KeSMSw4sVIPMDSecRwRtStLgrstOtwdInwdPos_175_Val/1 -> Terminator_72/1
  PA_KeSMSw4sVIPMDSecRwRtStLgrstOtwdInwdPos_180_Val/1 -> Terminator_73/1
  PA_KeSMSw4sVIPMDSecRwRtStLgrstOtwdInwdPos_Below160_Val/1 -> Terminator_74/1
  PA_KeSMSw4sVIPMDSecRwRtStLgrstOtwdInwdPos_Over180_Val/1 -> Terminator_75/1
  PA_KeSMSw6sAcsEntrySecRwRtStLgrstInwdOtwdPosMax_Val/1 -> Terminator_76/1
  PA_KeSMSw6sAcsEntrySecRwRtStLgrstInwdOtwdPosMin_Val/1 -> Terminator_77/1
  PA_KeSMSw6sAcsEntrySecRwRtStLgrstInwdOtwdPos_Val/1 -> Terminator_78/1
  PA_KeSMSw6sRecoveryMdSecRwRtStLgrstInwdOtwdPosMax_Val/1 -> Terminator_79/1
  PA_KeSMSw6sRecoveryMdSecRwRtStLgrstInwdOtwdPos_Val/1 -> Terminator_80/1
  PA_KeSMSwAcsEntrySecRwRtStLgrstInwdOtwdPosMax_Val/1 -> Terminator_81/1
  PA_KeSMSwAcsEntrySecRwRtStLgrstInwdOtwdPosMin_Val/1 -> Terminator_82/1
  PA_KeSMSwAcsEntrySecRwRtStLgrstInwdOtwdPos_Val/1 -> Terminator_83/1
  PA_KeSMSwRecovery6sMdSecRwRtStLgrstInwdOtwdPosMin_Val/1 -> Terminator_84/1
  PA_KeSMSwRecoveryMdSecRwRtStLgrstInwdOtwdPosMax_Val/1 -> Terminator_85/1
  PA_KeSMSwRecoveryMdSecRwRtStLgrstInwdOtwdPosMin_Val/1 -> Terminator_86/1
  PA_KeSMSwRecoveryMdSecRwRtStLgrstInwdOtwdPos_Val/1 -> Terminator_87/1
  PA_KeSMSw6sRecoveryMdSecRwRtStLgrstInwdOtwdPosMin_Val/1 -> Terminator_88/1
  PA_KeSMSwVIPMdSecRwRtStLgrstInwdOtwdPosMax_Val/1 -> Terminator_89/1
  PA_KeSMSwVIPMdSecRwRtStLgrstInwdOtwdPosMin_Val/1 -> Terminator_90/1
  PA_KeSMSwVIPMdSecRwRtStLgrstInwdOtwdPos_Val/1 -> Terminator_91/1
  PA_KeSMSwAcsMd8SecRwRtStLgrstInwdOtwdPosMax_Val/1 -> Terminator_92/1
  PA_KeSMSwAcsMd8SecRwRtStLgrstInwdOtwdPosMin_Val/1 -> Terminator_93/1
  PA_KeSMSwAcsMd8SecRwRtStLgrstInwdOtwdPos_Val/1 -> Terminator_94/1
  PA_KeSMSwAcsMd9SecRwRtStLgrstInwdOtwdPosMax_Val/1 -> Terminator_95/1
  PA_KeSMSwAcsMd9SecRwRtStLgrstInwdOtwdPosMin_Val/1 -> Terminator_96/1
  PA_KeSMSwAcsMd9SecRwRtStLgrstInwdOtwdPos_Val/1 -> Terminator_97/1
  PA_KeSMSw6SVIPMdSecRwRtStLgrstInwdOtwdPosMax_Val/1 -> Terminator_98/1
  PA_KeSMSw6SVIPMdSecRwRtStLgrstInwdOtwdPosMin_Val/1 -> Terminator_99/1
  PA_KeSMSw6SVIPMdSecRwRtStLgrstInwdOtwdPos_Val/1 -> Terminator_100/1

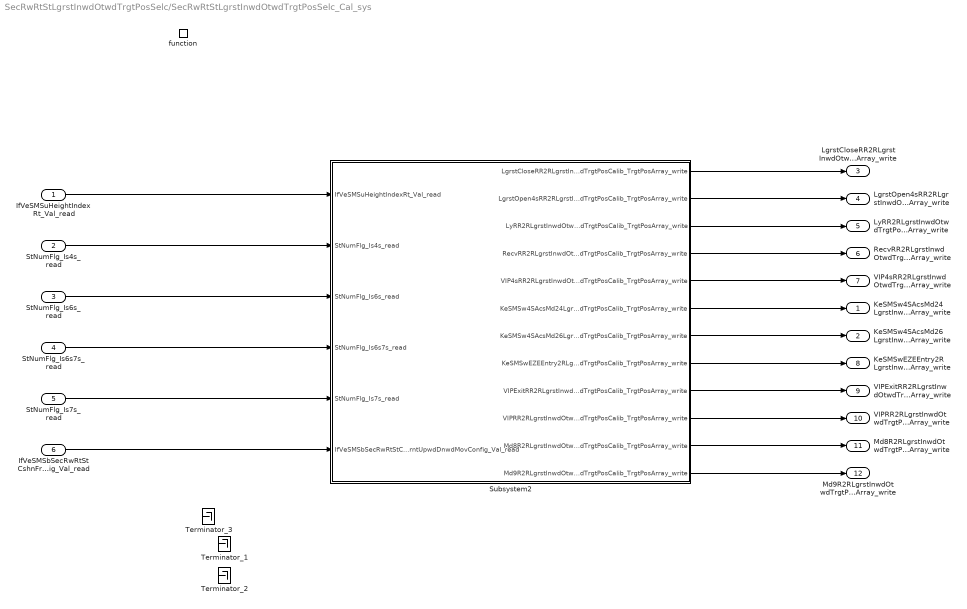
== system SecRwRtStLgrstInwdOtwdTrgtPosSelc/SecRwRtStLgrstInwdOtwdTrgtPosSelc_Cal_sys ==
  IfVeSMSuHeightIndexRt_Val_read : Inport
  StNumFlg_Is4s_read : Inport  Port=2
  StNumFlg_Is6s_read : Inport  Port=3
  StNumFlg_Is6s7s_read : Inport  Port=4
  StNumFlg_Is7s_read : Inport  Port=5
  IfVeSMSbSecRwRtStCshnFrntUpwdDnwdMovConfig_Val_read : Inport  Port=6
  function : TriggerPort  TriggerType=function-call  IsSimulinkFunction=on  FunctionName=SecRwRtStLgrstInwdOtwdTrgtPosSelc_Cal  VariantControl=(inherit)
  Subsystem2 : Subsystem
  Terminator_1 : Terminator
  Terminator_2 : Terminator
  Terminator_3 : Terminator
  KeSMSw4SAcsMd24LgrstInwdOtwdTrgtPosCalib_TrgtPosArray_write : Outport
      settings: EnsureOutportIsVirtual=on
  KeSMSw4SAcsMd26LgrstInwdOtwdTrgtPosCalib_TrgtPosArray_write : Outport  Port=2
      settings: EnsureOutportIsVirtual=on
  LgrstCloseRR2RLgrstInwdOtwdTrgtPosCalib_TrgtPosArray_write : Outport  Port=3
      settings: EnsureOutportIsVirtual=on
  LgrstOpen4sRR2RLgrstInwdOtwdTrgtPosCalib_TrgtPosArray_write : Outport  Port=4
      settings: EnsureOutportIsVirtual=on
  LyRR2RLgrstInwdOtwdTrgtPosCalib_TrgtPosArray_write : Outport  Port=5
      settings: EnsureOutportIsVirtual=on
  RecvRR2RLgrstInwdOtwdTrgtPosCalib_TrgtPosArray_write : Outport  Port=6
      settings: EnsureOutportIsVirtual=on
  VIP4sRR2RLgrstInwdOtwdTrgtPosCalib_TrgtPosArray_write : Outport  Port=7
      settings: EnsureOutportIsVirtual=on
  KeSMSwEZEEntry2RLgrstInwdOtwdTrgtPosCalib_TrgtPosArray_write : Outport  Port=8
      settings: EnsureOutportIsVirtual=on
  VIPExitRR2RLgrstInwdOtwdTrgtPosCalib_TrgtPosArray_write : Outport  Port=9
      settings: EnsureOutportIsVirtual=on
  VIPRR2RLgrstInwdOtwdTrgtPosCalib_TrgtPosArray_write : Outport  Port=10
      settings: EnsureOutportIsVirtual=on
  Md8R2RLgrstInwdOtwdTrgtPosCalib_TrgtPosArray_write : Outport  Port=11
      settings: EnsureOutportIsVirtual=on
  Md9R2RLgrstInwdOtwdTrgtPosCalib_TrgtPosArray_write : Outport  Port=12
      settings: EnsureOutportIsVirtual=on
  wires:
  Subsystem2/1(LgrstCloseRR2RLgrstInwdOtwdTrgtPosCalib_TrgtPosArray_write) -> LgrstCloseRR2RLgrstInwdOtwdTrgtPosCalib_TrgtPosArray_write/1
  Subsystem2/2(LgrstOpen4sRR2RLgrstInwdOtwdTrgtPosCalib_TrgtPosArray_write) -> LgrstOpen4sRR2RLgrstInwdOtwdTrgtPosCalib_TrgtPosArray_write/1
  Subsystem2/3(LyRR2RLgrstInwdOtwdTrgtPosCalib_TrgtPosArray_write) -> LyRR2RLgrstInwdOtwdTrgtPosCalib_TrgtPosArray_write/1
  Subsystem2/4(RecvRR2RLgrstInwdOtwdTrgtPosCalib_TrgtPosArray_write) -> RecvRR2RLgrstInwdOtwdTrgtPosCalib_TrgtPosArray_write/1
  Subsystem2/5(VIP4sRR2RLgrstInwdOtwdTrgtPosCalib_TrgtPosArray_write) -> VIP4sRR2RLgrstInwdOtwdTrgtPosCalib_TrgtPosArray_write/1
  Subsystem2/6(KeSMSw4SAcsMd24LgrstInwdOtwdTrgtPosCalib_TrgtPosArray_write) -> KeSMSw4SAcsMd24LgrstInwdOtwdTrgtPosCalib_TrgtPosArray_write/1
  Subsystem2/7(KeSMSw4SAcsMd26LgrstInwdOtwdTrgtPosCalib_TrgtPosArray_write) -> KeSMSw4SAcsMd26LgrstInwdOtwdTrgtPosCalib_TrgtPosArray_write/1
  IfVeSMSuHeightIndexRt_Val_read/1 -> Subsystem2/1(IfVeSMSuHeightIndexRt_Val_read)
  StNumFlg_Is4s_read/1 -> Subsystem2/2(StNumFlg_Is4s_read)
  StNumFlg_Is6s_read/1 -> Subsystem2/3(StNumFlg_Is6s_read)
  StNumFlg_Is6s7s_read/1 -> Subsystem2/4(StNumFlg_Is6s7s_read)
  StNumFlg_Is7s_read/1 -> Subsystem2/5(StNumFlg_Is7s_read)
  Subsystem2/8(KeSMSwEZEEntry2RLgrstInwdOtwdTrgtPosCalib_TrgtPosArray_write) -> KeSMSwEZEEntry2RLgrstInwdOtwdTrgtPosCalib_TrgtPosArray_write/1
  IfVeSMSbSecRwRtStCshnFrntUpwdDnwdMovConfig_Val_read/1 -> Subsystem2/6(IfVeSMSbSecRwRtStCshnFrntUpwdDnwdMovConfig_Val_read)
  Subsystem2/10(VIPRR2RLgrstInwdOtwdTrgtPosCalib_TrgtPosArray_write) -> VIPRR2RLgrstInwdOtwdTrgtPosCalib_TrgtPosArray_write/1
  Subsystem2/9(VIPExitRR2RLgrstInwdOtwdTrgtPosCalib_TrgtPosArray_write) -> VIPExitRR2RLgrstInwdOtwdTrgtPosCalib_TrgtPosArray_write/1
  Subsystem2/11(Md8R2RLgrstInwdOtwdTrgtPosCalib_TrgtPosArray_write) -> Md8R2RLgrstInwdOtwdTrgtPosCalib_TrgtPosArray_write/1
  Subsystem2/12(Md9R2RLgrstInwdOtwdTrgtPosCalib_TrgtPosArray_write) -> Md9R2RLgrstInwdOtwdTrgtPosCalib_TrgtPosArray_write/1
  ? -> Terminator_1/1
  ? -> Terminator_2/1
  ? -> Terminator_3/1

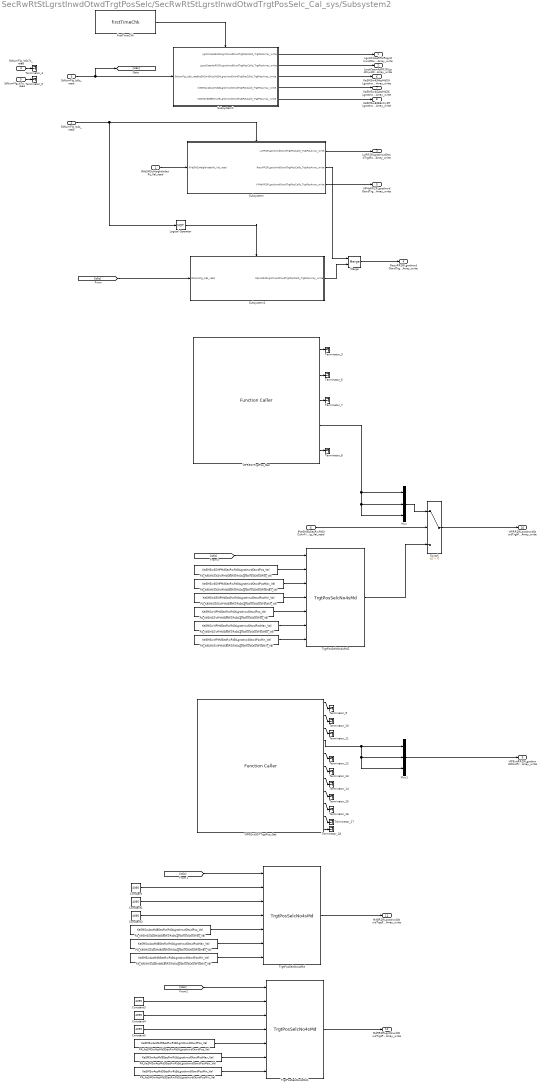
== system SecRwRtStLgrstInwdOtwdTrgtPosSelc/SecRwRtStLgrstInwdOtwdTrgtPosSelc_Cal_sys/Subsystem2 ==
  IfVeSMSuHeightIndexRt_Val_read : Inport
  StNumFlg_Is4s_read : Inport  Port=2
  StNumFlg_Is6s_read : Inport  Port=3
  StNumFlg_Is6s7s_read : Inport  Port=4
  StNumFlg_Is7s_read : Inport  Port=5
  IfVeSMSbSecRwRtStCshnFrntUpwdDnwdMovConfig_Val_read : Inport  Port=6
  Constant{,1..5} (6 alike) : Constant  Value=4095  OutDataTypeStr=uint16
  Logical Operator : Logic  Operator=NOT  AllPortsSameDT=off  OutDataTypeStr=boolean
  Merge : Merge
  Mux : Mux  Inputs=3
  Mux1 : Mux  Inputs=3
  PA_KeSMSw6SVIPMdSecRwRtStLgrstInwdOtwdPosMax_Val : Constant  Value=KeSMSw6SVIPMdSecRwRtStLgrstInwdOtwdPosMax_Val
  PA_KeSMSw6SVIPMdSecRwRtStLgrstInwdOtwdPosMin_Val : Constant  Value=KeSMSw6SVIPMdSecRwRtStLgrstInwdOtwdPosMin_Val
  PA_KeSMSw6SVIPMdSecRwRtStLgrstInwdOtwdPos_Val : Constant  Value=KeSMSw6SVIPMdSecRwRtStLgrstInwdOtwdPos_Val
  PA_KeSMSwAcsMd8SecRwRtStLgrstInwdOtwdPosMax_Val : Constant  Value=KeSMSwAcsMd8SecRwRtStLgrstInwdOtwdPosMax_Val
  PA_KeSMSwAcsMd8SecRwRtStLgrstInwdOtwdPosMin_Val : Constant  Value=KeSMSwAcsMd8SecRwRtStLgrstInwdOtwdPosMin_Val
  PA_KeSMSwAcsMd8SecRwRtStLgrstInwdOtwdPos_Val : Constant  Value=KeSMSwAcsMd8SecRwRtStLgrstInwdOtwdPos_Val
  PA_KeSMSwAcsMd9SecRwRtStLgrstInwdOtwdPosMax_Val : Constant  Value=KeSMSwAcsMd9SecRwRtStLgrstInwdOtwdPosMax_Val
  PA_KeSMSwAcsMd9SecRwRtStLgrstInwdOtwdPosMin_Val : Constant  Value=KeSMSwAcsMd9SecRwRtStLgrstInwdOtwdPosMin_Val
  PA_KeSMSwAcsMd9SecRwRtStLgrstInwdOtwdPos_Val : Constant  Value=KeSMSwAcsMd9SecRwRtStLgrstInwdOtwdPos_Val
  PA_KeSMSwVIPMdSecRwRtStLgrstInwdOtwdPosMax_Val : Constant  Value=KeSMSwVIPMdSecRwRtStLgrstInwdOtwdPosMax_Val
  PA_KeSMSwVIPMdSecRwRtStLgrstInwdOtwdPosMin_Val : Constant  Value=KeSMSwVIPMdSecRwRtStLgrstInwdOtwdPosMin_Val
  PA_KeSMSwVIPMdSecRwRtStLgrstInwdOtwdPos_Val : Constant  Value=KeSMSwVIPMdSecRwRtStLgrstInwdOtwdPos_Val
  Subsystem : Subsystem
  Subsystem1 : Subsystem
  Subsystem2 : Subsystem
  Switch : Switch  Criteria=u2 > Threshold
  Terminator_{3..18} (16 alike) : Terminator
  TrgtPosSelcNo4sMd : TrgtPosSelcLib/TrgtPosSelcNo4sMd  SystemSampleTime=-1
  TrgtPosSelcNo4sMd1 : TrgtPosSelcLib/TrgtPosSelcNo4sMd  SystemSampleTime=-1
  TrgtPosSelcNo4sMd2 : TrgtPosSelcLib/TrgtPosSelcNo4sMd  SystemSampleTime=-1
  VIPR557TrgtPos_Get : FunctionCaller  FunctionPrototype=[SecRwLtStBkReclnTrgtPos,SecRwLtStZeroTrgtPos,SecRwLtStLgrstUpwdDnwdTrgtPos,SecRwLtStLgrstInwdOtwdTrgtPos,SecRwLtStFwdBkwdTrgtPos] = VIPR557TrgtPos_Get()  OutputArgumentSpecifications=uint16(1), uint16(1), uint16(1), uint16(1), uint16(1)
  VIPRExit557TrgtPos_Get : FunctionCaller  FunctionPrototype=[SecRwRtStBkReclnTrgtPos,SecRwRtStZeroTrgtPos,SecRwRtStLgrstUpwdDnwdTrgtPos,SecRwRtStLgrstInwdOtwdTrgtPos,ThdRwLtStBkReclnTrgtPos,ThdRwLtStFwdBkwdTrgtPos,ThdRwRtStBkReclnTrgtPos,ThdRwRtStFwdBkwdTrgtPos,PassStBkReclnTrgtPos,PassStFwdBkwdTrgtPos,SecRwRtStFwdBkwdTrgtPos] = VIPRExit557TrgtPos_Get()  OutputArgumentSpecifications=uint16(1), uint16(1), uint16(1), uint16(1), uint16(1), uint16(1), uint16(1), uint16(1), uint16(1), uint16(1), uint16(1)
  firstTimeChk : TrgtPosSelcLib/firstTimeChk  SystemSampleTime=-1
  LgrstCloseRR2RLgrstInwdOtwdTrgtPosCalib_TrgtPosArray_write : Outport
      settings: EnsureOutportIsVirtual=on
  LgrstOpen4sRR2RLgrstInwdOtwdTrgtPosCalib_TrgtPosArray_write : Outport  Port=2
      settings: EnsureOutportIsVirtual=on
  LyRR2RLgrstInwdOtwdTrgtPosCalib_TrgtPosArray_write : Outport  Port=3
      settings: EnsureOutportIsVirtual=on
  RecvRR2RLgrstInwdOtwdTrgtPosCalib_TrgtPosArray_write : Outport  Port=4
      settings: EnsureOutportIsVirtual=on
  VIP4sRR2RLgrstInwdOtwdTrgtPosCalib_TrgtPosArray_write : Outport  Port=5
      settings: EnsureOutportIsVirtual=on
  KeSMSw4SAcsMd24LgrstInwdOtwdTrgtPosCalib_TrgtPosArray_write : Outport  Port=6
      settings: EnsureOutportIsVirtual=on
  KeSMSw4SAcsMd26LgrstInwdOtwdTrgtPosCalib_TrgtPosArray_write : Outport  Port=7
      settings: EnsureOutportIsVirtual=on
  KeSMSwEZEEntry2RLgrstInwdOtwdTrgtPosCalib_TrgtPosArray_write : Outport  Port=8
      settings: EnsureOutportIsVirtual=on
  VIPExitRR2RLgrstInwdOtwdTrgtPosCalib_TrgtPosArray_write : Outport  Port=9
      settings: EnsureOutportIsVirtual=on
  VIPRR2RLgrstInwdOtwdTrgtPosCalib_TrgtPosArray_write : Outport  Port=10
      settings: EnsureOutportIsVirtual=on
  Md8R2RLgrstInwdOtwdTrgtPosCalib_TrgtPosArray_write : Outport  Port=11
      settings: EnsureOutportIsVirtual=on
  Md9R2RLgrstInwdOtwdTrgtPosCalib_TrgtPosArray_write : Outport  Port=12
      settings: EnsureOutportIsVirtual=on
  wires:
  Subsystem/1(LyRR2RLgrstInwdOtwdTrgtPosCalib_TrgtPosArray_write) -> LyRR2RLgrstInwdOtwdTrgtPosCalib_TrgtPosArray_write/1
  firstTimeChk/1 -> Subsystem1/Enable
  StNumFlg_Is6s7s_read/1 -> Terminator_4/1
  IfVeSMSuHeightIndexRt_Val_read/1 -> Subsystem/1(IfVeSMSuHeightIndexRt_Val_read)
  StNumFlg_Is7s_read/1 -> Terminator_5/1
  Subsystem/3(VIP4sRR2RLgrstInwdOtwdTrgtPosCalib_TrgtPosArray_write) -> VIP4sRR2RLgrstInwdOtwdTrgtPosCalib_TrgtPosArray_write/1
  Subsystem1/1(LgrstCloseRR2RLgrstInwdOtwdTrgtPosCalib_TrgtPosArray_write) -> LgrstCloseRR2RLgrstInwdOtwdTrgtPosCalib_TrgtPosArray_write/1
  Subsystem1/2(LgrstOpen4sRR2RLgrstInwdOtwdTrgtPosCalib_TrgtPosArray_write) -> LgrstOpen4sRR2RLgrstInwdOtwdTrgtPosCalib_TrgtPosArray_write/1
  StNumFlg_Is4s_read/1 -> Logical Operator/1, Subsystem/Enable
  Subsystem1/4(KeSMSw4SAcsMd26LgrstInwdOtwdTrgtPosCalib_TrgtPosArray_write) -> KeSMSw4SAcsMd26LgrstInwdOtwdTrgtPosCalib_TrgtPosArray_write/1
  Subsystem1/3(KeSMSw4SAcsMd24LgrstInwdOtwdTrgtPosCalib_TrgtPosArray_write) -> KeSMSw4SAcsMd24LgrstInwdOtwdTrgtPosCalib_TrgtPosArray_write/1
  Subsystem1/5(KeSMSwEZEEntry2RLgrstInwdOtwdTrgtPosCalib_TrgtPosArray_write) -> KeSMSwEZEEntry2RLgrstInwdOtwdTrgtPosCalib_TrgtPosArray_write/1
  StNumFlg_Is6s_read/1 -> [is6s], Subsystem1/1(StNumFlg_Is6s_read)
  [is6s] -> Subsystem2/1(StNumFlg_Is6s_read)
  Logical Operator/1 -> Subsystem2/Enable
  Subsystem2/1(RecvRR2RLgrstInwdOtwdTrgtPosCalib_TrgtPosArray_write) -> Merge/2
  Merge/1 -> RecvRR2RLgrstInwdOtwdTrgtPosCalib_TrgtPosArray_write/1
  Subsystem/2(RecvRR2RLgrstInwdOtwdTrgtPosCalib_TrgtPosArray_write) -> Merge/1
  IfVeSMSbSecRwRtStCshnFrntUpwdDnwdMovConfig_Val_read/1 -> Switch/2
  Mux/1 -> Switch/1
  VIPR557TrgtPos_Get/4 -> Mux/3, Mux/2, Mux/1
  Switch/1 -> VIPRR2RLgrstInwdOtwdTrgtPosCalib_TrgtPosArray_write/1
  VIPRExit557TrgtPos_Get/4 -> Mux1/3, Mux1/2, Mux1/1
  Mux1/1 -> VIPExitRR2RLgrstInwdOtwdTrgtPosCalib_TrgtPosArray_write/1
  VIPR557TrgtPos_Get/1 -> Terminator_3/1
  VIPR557TrgtPos_Get/2 -> Terminator_6/1
  VIPR557TrgtPos_Get/3 -> Terminator_7/1
  VIPR557TrgtPos_Get/5 -> Terminator_8/1
  VIPRExit557TrgtPos_Get/1 -> Terminator_9/1
  VIPRExit557TrgtPos_Get/2 -> Terminator_10/1
  VIPRExit557TrgtPos_Get/3 -> Terminator_11/1
  VIPRExit557TrgtPos_Get/5 -> Terminator_12/1
  VIPRExit557TrgtPos_Get/6 -> Terminator_13/1
  VIPRExit557TrgtPos_Get/7 -> Terminator_14/1
  VIPRExit557TrgtPos_Get/8 -> Terminator_15/1
  VIPRExit557TrgtPos_Get/9 -> Terminator_16/1
  VIPRExit557TrgtPos_Get/10 -> Terminator_17/1
  VIPRExit557TrgtPos_Get/11 -> Terminator_18/1
  TrgtPosSelcNo4sMd/1 -> Md8R2RLgrstInwdOtwdTrgtPosCalib_TrgtPosArray_write/1
  TrgtPosSelcNo4sMd1/1 -> Md9R2RLgrstInwdOtwdTrgtPosCalib_TrgtPosArray_write/1
  [is6s] -> TrgtPosSelcNo4sMd/1
  [is6s] -> TrgtPosSelcNo4sMd1/1
  PA_KeSMSwAcsMd8SecRwRtStLgrstInwdOtwdPos_Val/1 -> TrgtPosSelcNo4sMd/5
  PA_KeSMSwAcsMd8SecRwRtStLgrstInwdOtwdPosMax_Val/1 -> TrgtPosSelcNo4sMd/6
  PA_KeSMSwAcsMd8SecRwRtStLgrstInwdOtwdPosMin_Val/1 -> TrgtPosSelcNo4sMd/7
  Constant/1 -> TrgtPosSelcNo4sMd/2
  Constant1/1 -> TrgtPosSelcNo4sMd/3
  Constant2/1 -> TrgtPosSelcNo4sMd/4
  Constant5/1 -> TrgtPosSelcNo4sMd1/4
  Constant4/1 -> TrgtPosSelcNo4sMd1/3
  Constant3/1 -> TrgtPosSelcNo4sMd1/2
  PA_KeSMSwAcsMd9SecRwRtStLgrstInwdOtwdPos_Val/1 -> TrgtPosSelcNo4sMd1/5
  PA_KeSMSwAcsMd9SecRwRtStLgrstInwdOtwdPosMax_Val/1 -> TrgtPosSelcNo4sMd1/6
  PA_KeSMSwAcsMd9SecRwRtStLgrstInwdOtwdPosMin_Val/1 -> TrgtPosSelcNo4sMd1/7
  TrgtPosSelcNo4sMd2/1 -> Switch/3
  [is6s] -> TrgtPosSelcNo4sMd2/1
  PA_KeSMSw6SVIPMdSecRwRtStLgrstInwdOtwdPosMax_Val/1 -> TrgtPosSelcNo4sMd2/3
  PA_KeSMSw6SVIPMdSecRwRtStLgrstInwdOtwdPos_Val/1 -> TrgtPosSelcNo4sMd2/2
  PA_KeSMSw6SVIPMdSecRwRtStLgrstInwdOtwdPosMin_Val/1 -> TrgtPosSelcNo4sMd2/4
  PA_KeSMSwVIPMdSecRwRtStLgrstInwdOtwdPosMax_Val/1 -> TrgtPosSelcNo4sMd2/6
  PA_KeSMSwVIPMdSecRwRtStLgrstInwdOtwdPos_Val/1 -> TrgtPosSelcNo4sMd2/5
  PA_KeSMSwVIPMdSecRwRtStLgrstInwdOtwdPosMin_Val/1 -> TrgtPosSelcNo4sMd2/7
